simulink model "prob1"  (R2015a)
settings: Solver=ode45  StartTime=0.0  StopTime=10.0  RelTol=1e-3
settings Model: Creator=Timothy  LastModifiedBy=Timothy

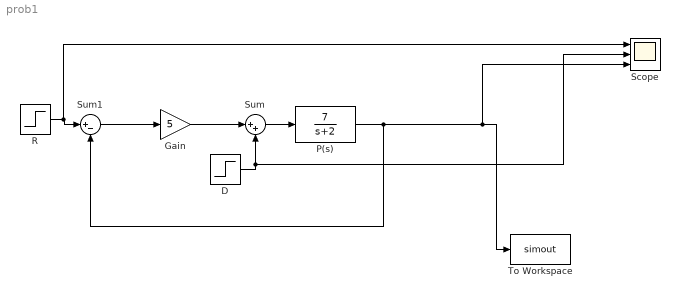
== system prob1 ==
  D : Step  After=-1  SampleTime=0
  Gain : Gain  Gain=5
  P(s) : TransferFcn  Numerator=[7]  Denominator=[1 2]
  R : Step  After=3  SampleTime=0
  Scope : Scope  NumInputPorts=3
      settings: YMin=-5~-5~-5  YMax=5~5~5
  Sum : Sum  Inputs=|++
  Sum1 : Sum  Inputs=|+-
  To Workspace : ToWorkspace  VariableName=simout  SaveFormat=Timeseries  SampleTime=-1
  wires:
  Sum/1 -> P(s)/1
  Gain/1 -> Sum/1
  Sum1/1 -> Gain/1
  R/1 -> Scope/1, Sum1/1
  P(s)/1 -> Scope/3, To Workspace/1, Sum1/2
  D/1 -> Scope/2, Sum/2
